simulink subsystem "HIL"  (R2024a)
settings: Solver=VariableStepAuto  StartTime=0.0  StopTime=10.0  RelTol=1e-3
values from neighbouring files (symbols this model uses):
  Hil = 100.0    [ModelDD.sldd]
  Sim : value not decoded    [ModelDD.sldd]
undefined symbols (not defined in the file or in its folder): D1, Delta, DiscIntNeverNeededParam
libraries: simulink x60, spsSeriesRLCBranchLib x18, spsControlledVoltageSourceLib x15, spsThreePhaseVIMeasurementLib x9, spsGroundLib x8, hdlsllib x6, spsMosfetLib x6, spsabctodq0Lib x5, spsDCVoltageSourceLib x3, spsPower3phInstantaneousLib x3, spsVoltageMeasurementLib x3, spspowerguiLib x3
(part 2 of 3)

== system HIL/PWM/Average ==
  DutyIn : Inport
  Iabc : Inport  Port=2
  Bias : Bias  Bias=0.5  SaturateOnIntegerOverflow=off
  Compare To Constant : simulink/Logic and Bit Operations/Compare To Constant  relop=>=  const=single(1.2)  OutDataTypeStr=boolean
  Compare To Constant1 : simulink/Logic and Bit Operations/Compare To Constant  relop=<=  const=single(0.8)  OutDataTypeStr=boolean
  Gain : Gain  Gain=-1
  Manual Switch : ManualSwitch  CurrentSetting=0
  OR : Logic  Operator=NOR  IconShape=distinctive  AllPortsSameDT=off  OutDataTypeStr=boolean
  PID Controller : slpidlib/PID Controller  Controller=PI  Form=Parallel  TimeDomain=Discrete-time  UseExternalTs=off  SampleTime=-1  IntegratorMethod=Forward Euler  FilterMethod=Forward Euler  ControllerParametersSource=internal  P=30*2/Hil.HVDC_V  I=(2*pi*4000)*30*2/Hil.HVDC_V  UseKiTs=off  D=0  UseExternalDerivativeSource=off  N=100  UseFilter=on  TunerSelectOption=Transfer Function Based (PID Tuner App)  InitialConditionSource=internal  InitialConditionForIntegrator=0  InitialConditionForFilter=0  DifferentiatorICPrevScaledInput=0  ExternalReset=none  TrackingMode=off  Kt=1  LimitOutput=on  SatLimitsSource=internal  UpperSaturationLimit=0.5  LowerSaturationLimit=-0.5  LinearizeAsGain=on  AntiWindupMode=clamping  Kb=1  LimitIntegrator=off  UpperIntegratorSaturationLimit=inf  LowerIntegratorSaturationLimit=-inf  POutMin=[]  POutMax=[]  IOutMin=[]  IOutMax=[]  DOutMin=[]  DOutMax=[]  NOutMin=[]  NOutMax=[]  SumOutMin=[]  SumOutMax=[]  SaturationOutMin=[]  SaturationOutMax=[]  PParamMin=[]  PParamMax=[]  IParamMin=[]  IParamMax=[]  DParamMin=[]  DParamMax=[]  NParamMin=[]  NParamMax=[]  KbParamMin=[]  KbParamMax=[]  KtParamMin=[]  KtParamMax=[]  KbOutMin=[]  KbOutMax=[]  KtOutMin=[]  KtOutMax=[]  IntegratorOutMin=[]  IntegratorOutMax=[]  FilterOutMin=[]  FilterOutMax=[]  SumI1OutMin=[]  SumI1OutMax=[]  SumI2OutMin=[]  SumI2OutMax=[]  SumI3OutMin=[]  SumI3OutMax=[]  SumI4OutMin=[]  SumI4OutMax=[]  SumDOutMin=[]  SumDOutMax=[]  DifferentiatorOutMin=[]  DifferentiatorOutMax=[]  FilterDiffOutCoefMin=[]  FilterDiffOutCoefMax=[]  ReciprocalOutMin=[]  ReciprocalOutMax=[]  SumDenOutMin=[]  SumDenOutMax=[]  SumNumOutMin=[]  SumNumOutMax=[]  DivideOutMin=[]  DivideOutMax=[]  UdiffTsProdOutMin=[]  UdiffTsProdOutMax=[]  NTsProdOutMin=[]  NTsProdOutMax=[]  UintegralTsProdOutMin=[]  UintegralTsProdOutMax=[]  UngainTsProdOutMin=[]  UngainTsProdOutMax=[]  ClampingZeroOutDataTypeStr=Inherit: Inherit via back propagation  ClampingZeroOutMin=[]  ClampingZeroOutMax=[]  FilterDenConstantOutDataTypeStr=Inherit: Inherit via back propagation  FilterDenConstantOutMin=[]  FilterDenConstantOutMax=[]  PCopyOutDataTypeStr=Inherit: Inherit via back propagation  PCopyOutMin=[]  PCopyOutMax=[]  NCopyOutDataTypeStr=Inherit: Inherit via back propagation  NCopyOutMin=[]  NCopyOutMax=[]  IntegratorContinuousStateAttributes=''  IntegratorStateMustResolveToSignalObject=off  IntegratorRTWStateStorageClass=Auto  FilterContinuousStateAttributes=''  FilterStateMustResolveToSignalObject=off  FilterRTWStateStorageClass=Auto  ParallelPVariant=InternalParameters  IdealPVariant=Disabled  IVariant=InternalParameters  DVariant=Disabled  IntegratorVariant=Discrete  SatVariant=Enabled  AWVariant=DiscClampingParallel  PCopyVariant=Disabled  TRVariant=Disabled  FdbkBlocksVariant=Forward  IdealPFdbkVariant=Disabled  SatFdbkVariant=Disabled  DerivativeFilterVariant=Disabled  NVariant=Disabled  NCopyVariant=Disabled_SignalSpec  FilterICVariant=Disabled  IntegratorICVariant=InternalICs  ExternalResetVariant=Disabled  TRSumVariant=Passthrough  SumFdbkVariant=Disabled  SumVariant=Sum_PI  TsampFilterVariant=InternalTs  TsampNgainVariant=Passthrough  TsampIntegralVariant=Disabled_SignalSpec  ExternalSaturationOutDataTypeStr=Inherit: Same as second input  DerivativeSourceVariant=Disabled
  Relay : Relay  OffSwitchValue=-eps  OnOutputValue=0  OffOutputValue=1
  Selector : Selector  InputPortWidth=4  IndexOptions=Index vector (dialog)  Indices=[1 2 3]  OutputSizes=1
  Selector1 : Selector  InputPortWidth=4  IndexOptions=Index vector (dialog)  Indices=[1 4]  OutputSizes=1
  Sum of Elements : Sum  Inputs=+
  Switch : Switch  Criteria=u2 > Threshold  SaturateOnIntegerOverflow=off  InputSameDT=off
  PWMSix : Outport
  wires:
  Bias/1 -> Manual Switch/2
  PID Controller/1 -> Bias/1
  Manual Switch/1 -> Switch/3
  Gain/1 -> PID Controller/1
  OR/1 -> Switch/2
  Compare To Constant1/1 -> OR/2
  Iabc/1 -> Relay/1, Gain/1
  Switch/1 -> PWMSix/1
  Selector/1 -> Switch/1
  Relay/1 -> Manual Switch/1
  DutyIn/1 -> Selector1/1, Selector/1  "HIL_PWM"
  Selector1/1 -> Sum of Elements/1
  Sum of Elements/1 -> Compare To Constant/1, Compare To Constant1/1
  Compare To Constant/1 -> OR/1

== system HIL/PWM/PWM ==
  DutyIn : Inport
  Compare To Constant : simulink/Logic and Bit Operations/Compare To Constant  relop=<=  const=0.5  OutDataTypeStr=boolean
  Constant : Constant  Value=round(1/(Hil.PWM_Freq*Sim.ContSampleTime))
  Constant1 : Constant  OutDataTypeStr=boolean
  Constant2 : Constant  Value=round(Hil.PWM_Deadtime/Sim.ContSampleTime)  OutDataTypeStr=uint32
  Gain2 : Gain  Gain=0.5  OutDataTypeStr=uint32
  NOT : Logic  Operator=NOT  IconShape=distinctive  AllPortsSameDT=off  OutDataTypeStr=boolean
  PWM Generator : Subsystem
  Product : Product
  Product1 : Product
  Selector2 : Selector  InputPortWidth=4  IndexOptions=Index vector (dialog)  Indices=[1 2 3]  OutputSizes=1
  Selector3 : Selector  InputPortWidth=4  IndexOptions=Index vector (dialog)  Indices=[1 4]  OutputSizes=1
  Sum of Elements : Sum  Inputs=+
  Unit Delay1 : UnitDelay  SampleTime=-1  HasFrameUpgradeWarning=on
  PWMSix : Outport
  Trig : Outport  Port=2
  wires:
  DutyIn/1 -> Selector2/1, Selector3/1  "DutyIn"
  Sum of Elements/1 -> Compare To Constant/1
  Selector3/1 -> Sum of Elements/1  "DutyIn"
  Selector2/1 -> Product/1  "DutyIn"
  Compare To Constant/1 -> Unit Delay1/1
  PWM Generator/1(S) -> Product1/2
  Gain2/1 -> PWM Generator/2(Period), Product/2
  Constant1/1 -> PWM Generator/3(Enable)
  Constant2/1 -> PWM Generator/4(DeadBand)
  Constant/1 -> Gain2/1
  Product/1 -> PWM Generator/1(DutyCnt)  "DutyCnt"
  PWM Generator/2(Trig) -> Trig/1
  Unit Delay1/1 -> NOT/1
  Product1/1 -> PWMSix/1
  NOT/1 -> Product1/1

== system HIL/Sensors/Delta ==
  Vabc_g : Inport
  Iabc : Inport  Port=2
  Vdc : Inport  Port=3
  Bias : Bias  Bias=Hil.ADC_CH0_PHY_OFFSET  SaturateOnIntegerOverflow=off
  Bias1 : Bias  Bias=Hil.ADC_CH1_PHY_OFFSET  SaturateOnIntegerOverflow=off
  Bias2 : Bias  Bias=Hil.ADC_CH2_PHY_OFFSET  SaturateOnIntegerOverflow=off
  Bias3 : Bias  Bias=Hil.ADC_CH3_PHY_OFFSET  SaturateOnIntegerOverflow=off
  Bias4 : Bias  Bias=Hil.ADC_CH4_PHY_OFFSET  SaturateOnIntegerOverflow=off
  Bias5 : Bias  Bias=Hil.ADC_CH5_PHY_OFFSET  SaturateOnIntegerOverflow=off
  Demux2 : Demux  Outputs=3
  Demux3 : Demux  Outputs=3
  Gain : Gain  Gain=1/Hil.ADC_CH0_PHY_Gain
  Gain1 : Gain  Gain=1/Hil.ADC_CH4_PHY_Gain
  Gain2 : Gain  Gain=1/Hil.ADC_CH1_PHY_Gain
  Gain3 : Gain  Gain=1/Hil.ADC_CH3_PHY_Gain
  Gain5 : Gain  Gain=1/Hil.ADC_CH2_PHY_Gain
  Gain6 : Gain  Gain=1/Hil.ADC_CH5_PHY_Gain
  Terminator : Terminator
  ADC1 : Outport
  ADC2 : Outport  Port=2
  ADC3 : Outport  Port=3
  ADC4 : Outport  Port=4
  ADC5 : Outport  Port=5
  ADC6 : Outport  Port=6
  wires:
  Gain1/1 -> Bias4/1
  Gain5/1 -> Bias2/1
  Demux2/2 -> Gain2/1
  Demux2/1 -> Gain/1
  Gain6/1 -> Bias5/1
  Gain/1 -> Bias/1
  Demux3/1 -> Gain5/1
  Demux3/3 -> Gain1/1
  Gain3/1 -> Bias3/1
  Bias5/1 -> ADC6/1  "V_hvdc_5v"
  Bias1/1 -> ADC2/1  "V_Grid_b_5v"
  Demux3/2 -> Gain3/1
  Gain2/1 -> Bias1/1
  Iabc/1 -> Demux3/1
  Vabc_g/1 -> Demux2/1
  Bias/1 -> ADC1/1  "V_Grid_a_5v"
  Bias4/1 -> ADC5/1  "I_inv_b_5v"
  Bias2/1 -> ADC3/1  "V_Grid_c_5v"
  Vdc/1 -> Gain6/1
  Bias3/1 -> ADC4/1  "I_inv_a_5v"
  Demux2/3 -> Terminator/1

== system HIL/Sensors/Star ==
  Vabc_g : Inport
  Iabc : Inport  Port=2
  Vdc : Inport  Port=3
  Bias : Bias  Bias=Hil.ADC_CH0_PHY_OFFSET  SaturateOnIntegerOverflow=off
  Bias1 : Bias  Bias=Hil.ADC_CH1_PHY_OFFSET  SaturateOnIntegerOverflow=off
  Bias2 : Bias  Bias=Hil.ADC_CH2_PHY_OFFSET  SaturateOnIntegerOverflow=off
  Bias3 : Bias  Bias=Hil.ADC_CH3_PHY_OFFSET  SaturateOnIntegerOverflow=off
  Bias4 : Bias  Bias=Hil.ADC_CH4_PHY_OFFSET  SaturateOnIntegerOverflow=off
  Bias5 : Bias  Bias=Hil.ADC_CH5_PHY_OFFSET  SaturateOnIntegerOverflow=off
  Demux2 : Demux  Outputs=3
  Demux3 : Demux  Outputs=3
  Gain : Gain  Gain=1/Hil.ADC_CH0_PHY_Gain
  Gain1 : Gain  Gain=1/Hil.ADC_CH4_PHY_Gain
  Gain2 : Gain  Gain=1/Hil.ADC_CH1_PHY_Gain
  Gain3 : Gain  Gain=1/Hil.ADC_CH3_PHY_Gain
  Gain5 : Gain  Gain=1/Hil.ADC_CH2_PHY_Gain
  Gain6 : Gain  Gain=1/Hil.ADC_CH5_PHY_Gain
  Terminator1 : Terminator
  ADC1 : Outport
  ADC2 : Outport  Port=2
  ADC3 : Outport  Port=3
  ADC4 : Outport  Port=4
  ADC5 : Outport  Port=5
  ADC6 : Outport  Port=6
  wires:
  Bias3/1 -> ADC4/1  "I_inv_a_5v"
  Vdc/1 -> Gain6/1
  Bias2/1 -> ADC3/1  "V_Grid_c_5v"
  Bias4/1 -> ADC5/1  "I_inv_b_5v"
  Bias/1 -> ADC1/1  "V_Grid_a_5v"
  Vabc_g/1 -> Demux2/1
  Iabc/1 -> Demux3/1
  Gain2/1 -> Bias1/1
  Demux3/3 -> Terminator1/1
  Demux3/1 -> Gain3/1
  Bias1/1 -> ADC2/1  "V_Grid_b_5v"
  Bias5/1 -> ADC6/1  "V_hvdc_5v"
  Gain3/1 -> Bias3/1
  Demux3/2 -> Gain1/1
  Demux2/3 -> Gain5/1
  Gain/1 -> Bias/1
  Gain6/1 -> Bias5/1
  Demux2/1 -> Gain/1
  Demux2/2 -> Gain2/1
  Gain5/1 -> Bias2/1
  Gain1/1 -> Bias4/1

== system HIL/EquivelentSimscape/Continous/Harmonics ==
  wt_abc : Inport
  Enable : EnablePort
  Cos1 : Trigonometry  Operator=cos
  Gain5 : Gain  Gain=Hil.Harm_Freq'  Multiplication=Matrix(K*u)
  Gain8 : Gain  Gain=(eye(3,3).*(Hil.Harm_Amp))  Multiplication=Matrix(K*u)
  Reshape : Reshape
  Reshape1 : Reshape  OutputDimensionality=Row vector (2-D)
  Sum of Elements : Sum  Inputs=+  CollapseMode=Specified dimension
  Harm : Outport
  wires:
  Reshape/1 -> Harm/1
  Gain8/1 -> Sum of Elements/1
  Cos1/1 -> Gain8/1
  Gain5/1 -> Cos1/1
  Reshape1/1 -> Gain5/1
  wt_abc/1 -> Reshape1/1
  Sum of Elements/1 -> Reshape/1

== system HIL/EquivelentSimscape/Continous/Phase2Line ==
  In1 : Inport
  Demux : Demux  Outputs=3
  Mux1 : Mux  Inputs=3
  Sum{,1..3} (4 alike) : Sum  Inputs=|+-
  Sum4 : Sum  Inputs=-+|
  Sum5 : Sum  Inputs=-+|
  Out1 : Outport
  wires:
  Sum2/1 -> Sum5/2, Sum3/2  "CA"
  Sum1/1 -> Sum4/2, Sum5/1  "BC"
  Sum4/1 -> Mux1/2  "BC-AB"
  Sum5/1 -> Mux1/3  "CA-BC"
  Mux1/1 -> Out1/1
  Sum3/1 -> Mux1/1  "AB-CA"
  Sum/1 -> Sum3/1, Sum4/1  "AB"
  Demux/1 -> Sum/1, Sum2/2  "A"
  Demux/2 -> Sum1/1, Sum/2  "B"
  In1/1 -> Demux/1
  Demux/3 -> Sum2/1, Sum1/2  "C"

== system HIL/EquivelentSimscape/Continous/Phase2Line1 ==
  In1 : Inport
  Demux : Demux  Outputs=3
  Mux1 : Mux  Inputs=3
  Sum{,1..3} (4 alike) : Sum  Inputs=|+-
  Sum4 : Sum  Inputs=-+|
  Sum5 : Sum  Inputs=-+|
  Out1 : Outport
  wires:
  Demux/3 -> Sum1/2, Sum2/1  "C"
  In1/1 -> Demux/1
  Demux/2 -> Sum/2, Sum1/1  "B"
  Demux/1 -> Sum2/2, Sum/1  "A"
  Sum/1 -> Sum4/1, Sum3/1  "AB"
  Sum3/1 -> Mux1/1  "AB-CA"
  Mux1/1 -> Out1/1
  Sum5/1 -> Mux1/3  "CA-BC"
  Sum4/1 -> Mux1/2  "BC-AB"
  Sum1/1 -> Sum5/1, Sum4/2  "BC"
  Sum2/1 -> Sum3/2, Sum5/2  "CA"

== system HIL/EquivelentSimscape/Continous/Rectifier1 ==
  Io : Inport
  Abs : Abs  SaturateOnIntegerOverflow=off
  Constant : Constant  Value=Hil.Grid_Frq
  Cos : Trigonometry  Operator=cos
  Discrete-Time Integrator : DiscreteIntegrator  gainval=single(1)  InitialCondition=single(311)  SampleTime=-1  ICPrevOutput=DiscIntNeverNeededParam  ICPrevScaledInput=DiscIntNeverNeededParam
  Gain : Gain  Gain=1/Hil.HVDC_C
  Gain1 : Gain  Gain=1/0.2
  Gain2 : Gain  Gain=2*pi
  Gain3 : Gain  Gain=Hil.Grid_VphRms*sqrt(2)
  Gain4 : Gain  Gain=Hil.HVDC_Cesr
  Gain5 : Gain  Gain=1/500
  Gain6 : Gain  Gain=Hil.HVDC_AutoTrnsN
  Saturation : Saturate  UpperLimit=inf  LowerLimit=0
  Sum : Sum  Inputs=|++
  Sum1 : Sum  Inputs=-+-
  Sum2 : Sum  Inputs=|+-
  Unit Delay1 : UnitDelay  InitialCondition=single(311)  SampleTime=-1  HasFrameUpgradeWarning=on
  Unit Delay2 : UnitDelay  SampleTime=-1  HasFrameUpgradeWarning=on
  WrappedIntegrator : Subsystem
  Vo : Outport
  wires:
  Gain6/1 -> Abs/1  "Vrec"
  Gain5/1 -> Sum1/3
  Gain4/1 -> Sum/2
  Discrete-Time Integrator/1 -> Sum/1
  Abs/1 -> Sum2/1  "Vrec"
  Sum/1 -> Vo/1, Unit Delay1/1  "Vdc"
  Sum1/1 -> Gain/1, Gain4/1  "Ic"
  Gain/1 -> Discrete-Time Integrator/1
  Unit Delay1/1 -> Sum2/2, Gain5/1
  Saturation/1 -> Sum1/2
  Unit Delay2/1 -> Sum1/1
  Io/1 -> Unit Delay2/1
  Sum2/1 -> Gain1/1
  Gain3/1 -> Gain6/1  "Vrec"
  Gain1/1 -> Saturation/1  "ir"
  WrappedIntegrator/1(wt) -> Cos/1  "wt"
  Gain2/1 -> WrappedIntegrator/1(w)  "w"
  Cos/1 -> Gain3/1
  Constant/1 -> Gain2/1  "f"

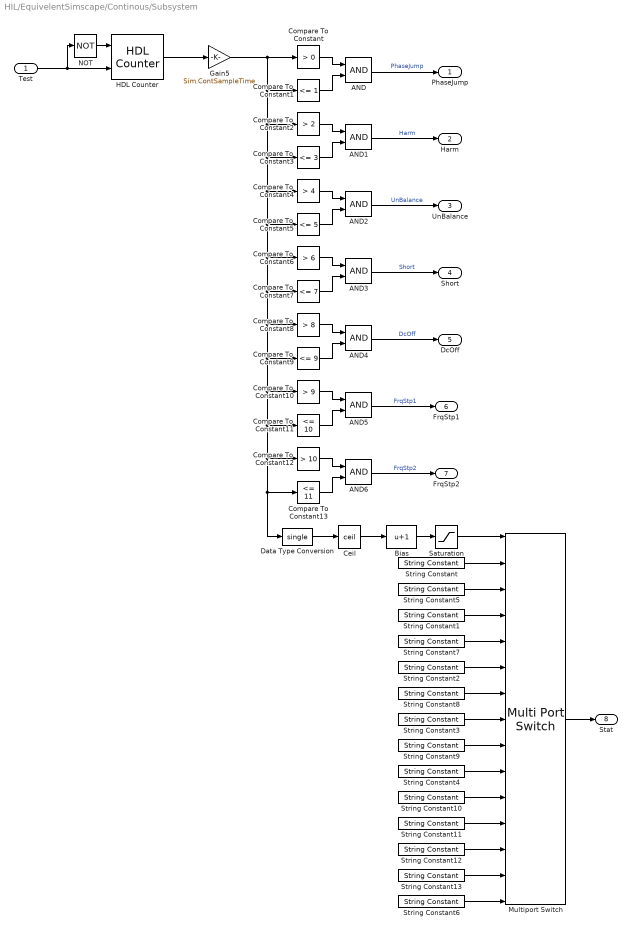
== system HIL/EquivelentSimscape/Continous/Subsystem ==
  Test : Inport
  AND{,1..6} (7 alike) : Logic  AllPortsSameDT=off  OutDataTypeStr=boolean
  Bias : Bias  Bias=1  SaturateOnIntegerOverflow=off
  Ceil : Rounding  Operator=ceil
  Compare To Constant : simulink/Logic and Bit Operations/Compare To Constant  relop=>  const=0  OutDataTypeStr=boolean
  Compare To Constant1 : simulink/Logic and Bit Operations/Compare To Constant  relop=<=  const=1  OutDataTypeStr=boolean
  Compare To Constant10 : simulink/Logic and Bit Operations/Compare To Constant  relop=>  const=9  OutDataTypeStr=boolean
  Compare To Constant11 : simulink/Logic and Bit Operations/Compare To Constant  relop=<=  const=10  OutDataTypeStr=boolean
  Compare To Constant12 : simulink/Logic and Bit Operations/Compare To Constant  relop=>  const=10  OutDataTypeStr=boolean
  Compare To Constant13 : simulink/Logic and Bit Operations/Compare To Constant  relop=<=  const=11  OutDataTypeStr=boolean
  Compare To Constant2 : simulink/Logic and Bit Operations/Compare To Constant  relop=>  const=2  OutDataTypeStr=boolean
  Compare To Constant3 : simulink/Logic and Bit Operations/Compare To Constant  relop=<=  const=3  OutDataTypeStr=boolean
  Compare To Constant4 : simulink/Logic and Bit Operations/Compare To Constant  relop=>  const=4  OutDataTypeStr=boolean
  Compare To Constant5 : simulink/Logic and Bit Operations/Compare To Constant  relop=<=  const=5  OutDataTypeStr=boolean
  Compare To Constant6 : simulink/Logic and Bit Operations/Compare To Constant  relop=>  const=6  OutDataTypeStr=boolean
  Compare To Constant7 : simulink/Logic and Bit Operations/Compare To Constant  relop=<=  const=7  OutDataTypeStr=boolean
  Compare To Constant8 : simulink/Logic and Bit Operations/Compare To Constant  relop=>  const=8  OutDataTypeStr=boolean
  Compare To Constant9 : simulink/Logic and Bit Operations/Compare To Constant  relop=<=  const=9  OutDataTypeStr=boolean
  Data Type Conversion : DataTypeConversion  OutDataTypeStr=single  SaturateOnIntegerOverflow=off  RndMeth=Floor
  Gain5 : Gain  Gain=Sim.ContSampleTime  ParamDataTypeStr=double  OutDataTypeStr=double
  HDL Counter : hdlsllib/Sources/HDL Counter  CountType=Free running  CountInit=0  CountStep=1  CountMax=25  CountFromType=Initial value  CountFrom=0  CountResetPort=on  CountLoadPort=off  CountEnbPort=on  CountDirPort=off  CountHitOutputPort=off  CountDataType=Unsigned  CountWordLen=32  CountFracLen=0  CountSampTime=1
  Multiport Switch : MultiPortSwitch  Inputs=14  SaturateOnIntegerOverflow=off  InputSameDT=off
  NOT : Logic  Operator=NOT  AllPortsSameDT=off  OutDataTypeStr=boolean
  Saturation : Saturate  UpperLimit=14  LowerLimit=0
  String Constant{,1..4,6,11} (7 alike) : StringConstant  String="\"Normal\""
  String Constant10 : StringConstant  String="\"DC Offset\""
  String Constant12 : StringConstant  String="\"Freq Stp 1\""
  String Constant13 : StringConstant  String="\"Freq Stp 2\""
  String Constant5 : StringConstant  String="\"Phase Jump\""
  String Constant7 : StringConstant  String="\"Harm\""
  String Constant8 : StringConstant  String="\"Unbalance\""
  String Constant9 : StringConstant  String="\"Short\""
  PhaseJump : Outport
  Harm : Outport  Port=2
  UnBalance : Outport  Port=3
  Short : Outport  Port=4
  DcOff : Outport  Port=5
  FrqStp1 : Outport  Port=6
  FrqStp2 : Outport  Port=7
  Stat : Outport  Port=8
  wires:
  Bias/1 -> Saturation/1
  Data Type Conversion/1 -> Ceil/1
  Multiport Switch/1 -> Stat/1
  Saturation/1 -> Multiport Switch/1
  Ceil/1 -> Bias/1
  String Constant13/1 -> Multiport Switch/14
  String Constant12/1 -> Multiport Switch/13
  String Constant11/1 -> Multiport Switch/12
  String Constant10/1 -> Multiport Switch/11
  String Constant9/1 -> Multiport Switch/9
  String Constant8/1 -> Multiport Switch/7
  String Constant7/1 -> Multiport Switch/5
  String Constant5/1 -> Multiport Switch/3
  String Constant6/1 -> Multiport Switch/15
  String Constant4/1 -> Multiport Switch/10
  String Constant3/1 -> Multiport Switch/8
  String Constant2/1 -> Multiport Switch/6
  String Constant1/1 -> Multiport Switch/4
  String Constant/1 -> Multiport Switch/2
  NOT/1 -> HDL Counter/1
  Compare To Constant13/1 -> AND6/2
  Compare To Constant12/1 -> AND6/1
  AND6/1 -> FrqStp2/1  "FrqStp2"
  AND5/1 -> FrqStp1/1  "FrqStp1"
  Compare To Constant10/1 -> AND5/1
  Compare To Constant11/1 -> AND5/2
  AND/1 -> PhaseJump/1  "PhaseJump"
  Test/1 -> HDL Counter/2, NOT/1
  AND2/1 -> UnBalance/1  "UnBalance"
  AND3/1 -> Short/1  "Short"
  HDL Counter/1 -> Gain5/1
  Compare To Constant5/1 -> AND2/2
  Compare To Constant/1 -> AND/1
  Compare To Constant9/1 -> AND4/2
  Compare To Constant2/1 -> AND1/1
  Compare To Constant8/1 -> AND4/1
  Compare To Constant3/1 -> AND1/2
  AND4/1 -> DcOff/1  "DcOff"
  Compare To Constant1/1 -> AND/2
  Compare To Constant7/1 -> AND3/2
  Compare To Constant6/1 -> AND3/1
  Gain5/1 -> Compare To Constant/1, Compare To Constant1/1, Compare To Constant3/1, Compare To Constant5/1, Compare To Constant7/1, Compare To Constant8/1, Compare To Constant9/1, Compare To Constant13/1, Data Type Conversion/1, Compare To Constant12/1, Compare To Constant11/1, Compare To Constant10/1, Compare To Constant6/1, Compare To Constant4/1, Compare To Constant2/1
  AND1/1 -> Harm/1  "Harm"
  Compare To Constant4/1 -> AND2/1

== system HIL/EquivelentSimscape/Continous/WrappedIntegrator ==
  w : Inport
  Constant1 : Constant  Value=2*pi
  Discrete-Time Integrator1 : DiscreteIntegrator  gainval=single(1)  ExternalReset=rising  InitialConditionSource=external  SampleTime=-1  ShowStatePort=on  ICPrevOutput=DiscIntNeverNeededParam  ICPrevScaledInput=DiscIntNeverNeededParam
  GreaterThan : RelationalOperator  Operator=~=  OutDataTypeStr=boolean  RndMeth=Simplest  InputSameDT=off
  Mod : Math  Operator=mod
  wt : Outport
  wires:
  GreaterThan/1 -> Discrete-Time Integrator1/2
  Discrete-Time Integrator1/1 -> wt/1  "wt"
  w/1 -> Discrete-Time Integrator1/1
  Discrete-Time Integrator1/State -> Mod/1, GreaterThan/1
  Mod/1 -> GreaterThan/2, Discrete-Time Integrator1/3
  Constant1/1 -> Mod/2

== system HIL/EquivelentSimscape/Continous/abc_dqz ==
  abc : Inport
  Ang : Inport  Port=2
  Subsystem : Subsystem
  Subsystem2 : Subsystem
  dqz : Outport  VectorParamsAs1DForOutWhenUnconnected=off
  wires:
  Subsystem2/1(dq) -> dqz/1
  Ang/1 -> Subsystem2/2(wtNow)
  Subsystem/1(al_be_0) -> Subsystem2/1(alpha_beta)
  abc/1 -> Subsystem/1(abc)

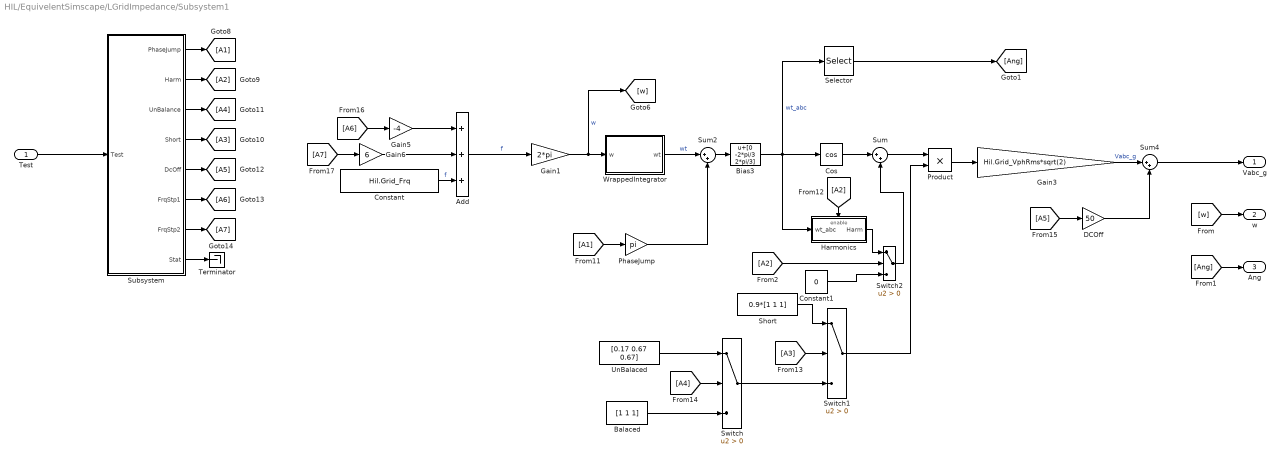
== system HIL/EquivelentSimscape/LGridImpedance/Subsystem1 ==
  Test : Inport
  Add : Sum  Inputs=+++
  Balaced : Constant  Value=[1 1 1]
  Bias3 : Bias  Bias=[0 -2*pi/3 2*pi/3]  SaturateOnIntegerOverflow=off
  Constant : Constant  Value=Hil.Grid_Frq
  Constant1 : Constant  Value=0
  Cos : Trigonometry  Operator=cos
  DCOff : Gain  Gain=50
  Gain1 : Gain  Gain=2*pi
  Gain3 : Gain  Gain=Hil.Grid_VphRms*sqrt(2)
  Gain5 : Gain  Gain=-4
  Gain6 : Gain  Gain=6
  Harmonics : Subsystem
  PhaseJump : Gain  Gain=pi
  Product : Product
  Selector : Selector  InputPortWidth=3  IndexOptions=Index vector (dialog)  Indices=[1]  OutputSizes=1
  Short : Constant  Value=0.9*[1 1 1]
  Subsystem : Subsystem
  Sum : Sum  Inputs=|++
  Sum2 : Sum  Inputs=|++
  Sum4 : Sum  Inputs=|++
  Switch : Switch  Criteria=u2 > Threshold  SaturateOnIntegerOverflow=off  InputSameDT=off
  Switch1 : Switch  Criteria=u2 > Threshold  SaturateOnIntegerOverflow=off  InputSameDT=off
  Switch2 : Switch  Criteria=u2 > Threshold  SaturateOnIntegerOverflow=off  InputSameDT=off
  Terminator : Terminator
  UnBalaced : Constant  Value=[0.17 0.67 0.67]
  WrappedIntegrator : Subsystem
  Vabc_g : Outport
  w : Outport  Port=2
  Ang : Outport  Port=3
  wires:
  [A2] -> Switch2/2
  Constant1/1 -> Switch2/3
  Harmonics/1(Harm) -> Switch2/1
  Subsystem/1(PhaseJump) -> [A1]
  [w] -> w/1
  [Ang] -> Ang/1
  Balaced/1 -> Switch/3
  Sum4/1 -> Vabc_g/1
  Test/1 -> Subsystem/1(Test)
  Cos/1 -> Sum/1
  Gain1/1 -> WrappedIntegrator/1(w), [w]  "w"
  Add/1 -> Gain1/1  "f"
  Selector/1 -> [Ang]
  PhaseJump/1 -> Sum2/2
  Gain3/1 -> Sum4/1  "Vabc_g"
  [A3] -> Switch1/2
  Subsystem/5(DcOff) -> [A5]
  Product/1 -> Gain3/1
  [A2] -> Harmonics/Enable
  Switch/1 -> Switch1/3
  Short/1 -> Switch1/1
  [A4] -> Switch/2
  Sum/1 -> Product/1
  Constant/1 -> Add/3  "f"
  Gain6/1 -> Add/2
  Subsystem/2(Harm) -> [A2]
  DCOff/1 -> Sum4/2
  Switch1/1 -> Product/2
  [A7] -> Gain6/1
  Subsystem/6(FrqStp1) -> [A6]
  WrappedIntegrator/1(wt) -> Sum2/1  "wt"
  Subsystem/8(Stat) -> Terminator/1
  [A6] -> Gain5/1
  UnBalaced/1 -> Switch/1
  Sum2/1 -> Bias3/1
  Gain5/1 -> Add/1
  [A5] -> DCOff/1
  Subsystem/7(FrqStp2) -> [A7]
  [A1] -> PhaseJump/1
  Bias3/1 -> Harmonics/1(wt_abc), Selector/1, Cos/1  "wt_abc"
  Switch2/1 -> Sum/2
  Subsystem/4(Short) -> [A3]
  Subsystem/3(UnBalance) -> [A4]

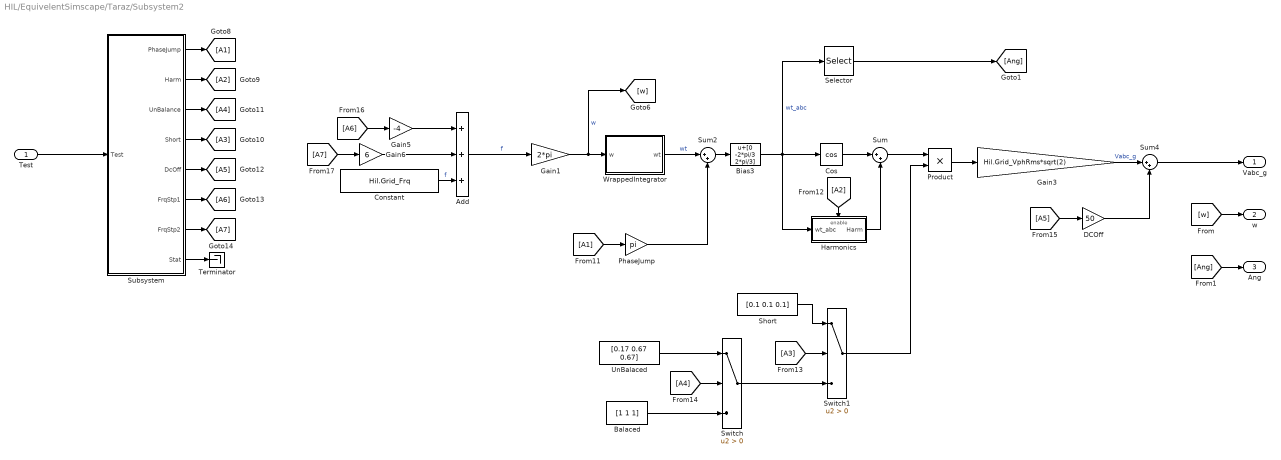
== system HIL/EquivelentSimscape/Taraz/Subsystem2 ==
  Test : Inport
  Add : Sum  Inputs=+++
  Balaced : Constant  Value=[1 1 1]
  Bias3 : Bias  Bias=[0 -2*pi/3 2*pi/3]  SaturateOnIntegerOverflow=off
  Constant : Constant  Value=Hil.Grid_Frq
  Cos : Trigonometry  Operator=cos
  DCOff : Gain  Gain=50
  Gain1 : Gain  Gain=2*pi
  Gain3 : Gain  Gain=Hil.Grid_VphRms*sqrt(2)
  Gain5 : Gain  Gain=-4
  Gain6 : Gain  Gain=6
  Harmonics : Subsystem
  PhaseJump : Gain  Gain=pi
  Product : Product
  Selector : Selector  InputPortWidth=3  IndexOptions=Index vector (dialog)  Indices=[1]  OutputSizes=1
  Short : Constant  Value=[0.1 0.1 0.1]
  Subsystem : Subsystem
  Sum : Sum  Inputs=|++
  Sum2 : Sum  Inputs=|++
  Sum4 : Sum  Inputs=|++
  Switch : Switch  Criteria=u2 > Threshold  SaturateOnIntegerOverflow=off  InputSameDT=off
  Switch1 : Switch  Criteria=u2 > Threshold  SaturateOnIntegerOverflow=off  InputSameDT=off
  Terminator : Terminator
  UnBalaced : Constant  Value=[0.17 0.67 0.67]
  WrappedIntegrator : Subsystem
  Vabc_g : Outport
  w : Outport  Port=2
  Ang : Outport  Port=3
  wires:
  Subsystem/1(PhaseJump) -> [A1]
  [w] -> w/1
  [Ang] -> Ang/1
  Balaced/1 -> Switch/3
  Sum4/1 -> Vabc_g/1
  Test/1 -> Subsystem/1(Test)
  Cos/1 -> Sum/1
  Gain1/1 -> WrappedIntegrator/1(w), [w]  "w"
  Add/1 -> Gain1/1  "f"
  Selector/1 -> [Ang]
  PhaseJump/1 -> Sum2/2
  Gain3/1 -> Sum4/1  "Vabc_g"
  [A3] -> Switch1/2
  Subsystem/5(DcOff) -> [A5]
  Product/1 -> Gain3/1
  [A2] -> Harmonics/Enable
  Switch/1 -> Switch1/3
  Short/1 -> Switch1/1
  [A4] -> Switch/2
  Sum/1 -> Product/1
  Constant/1 -> Add/3  "f"
  Gain6/1 -> Add/2
  Subsystem/2(Harm) -> [A2]
  DCOff/1 -> Sum4/2
  Switch1/1 -> Product/2
  [A7] -> Gain6/1
  Subsystem/6(FrqStp1) -> [A6]
  WrappedIntegrator/1(wt) -> Sum2/1  "wt"
  Subsystem/8(Stat) -> Terminator/1
  [A6] -> Gain5/1
  UnBalaced/1 -> Switch/1
  Sum2/1 -> Bias3/1
  Gain5/1 -> Add/1
  [A5] -> DCOff/1
  Subsystem/7(FrqStp2) -> [A7]
  [A1] -> PhaseJump/1
  Bias3/1 -> Harmonics/1(wt_abc), Selector/1, Cos/1  "wt_abc"
  Harmonics/1(Harm) -> Sum/2
  Subsystem/4(Short) -> [A3]
  Subsystem/3(UnBalance) -> [A4]

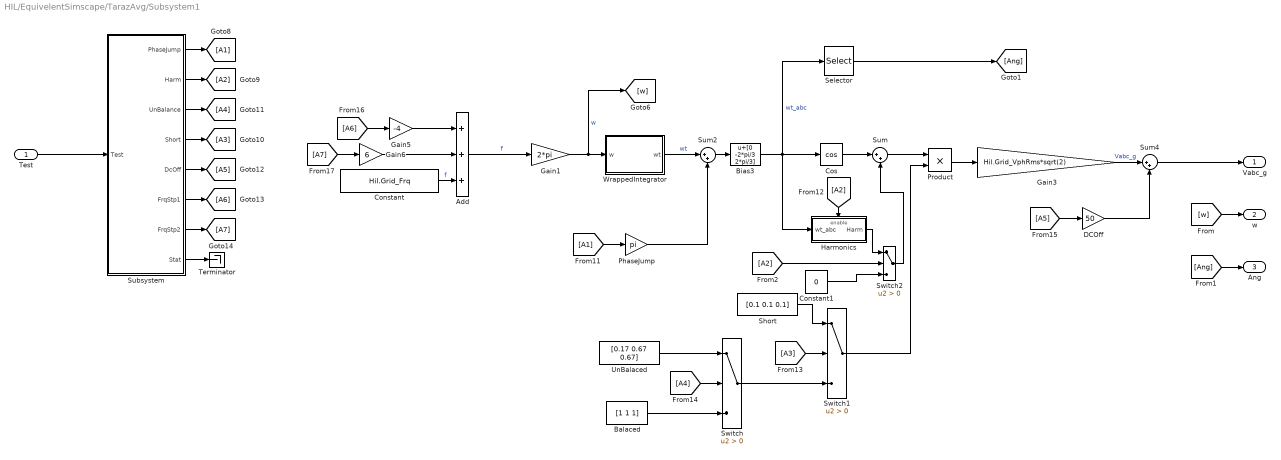
== system HIL/EquivelentSimscape/TarazAvg/Subsystem1 ==
  Test : Inport
  Add : Sum  Inputs=+++
  Balaced : Constant  Value=[1 1 1]
  Bias3 : Bias  Bias=[0 -2*pi/3 2*pi/3]  SaturateOnIntegerOverflow=off
  Constant : Constant  Value=Hil.Grid_Frq
  Constant1 : Constant  Value=0
  Cos : Trigonometry  Operator=cos
  DCOff : Gain  Gain=50
  Gain1 : Gain  Gain=2*pi
  Gain3 : Gain  Gain=Hil.Grid_VphRms*sqrt(2)
  Gain5 : Gain  Gain=-4
  Gain6 : Gain  Gain=6
  Harmonics : Subsystem
  PhaseJump : Gain  Gain=pi
  Product : Product
  Selector : Selector  InputPortWidth=3  IndexOptions=Index vector (dialog)  Indices=[1]  OutputSizes=1
  Short : Constant  Value=[0.1 0.1 0.1]
  Subsystem : Subsystem
  Sum : Sum  Inputs=|++
  Sum2 : Sum  Inputs=|++
  Sum4 : Sum  Inputs=|++
  Switch : Switch  Criteria=u2 > Threshold  SaturateOnIntegerOverflow=off  InputSameDT=off
  Switch1 : Switch  Criteria=u2 > Threshold  SaturateOnIntegerOverflow=off  InputSameDT=off
  Switch2 : Switch  Criteria=u2 > Threshold  SaturateOnIntegerOverflow=off  InputSameDT=off
  Terminator : Terminator
  UnBalaced : Constant  Value=[0.17 0.67 0.67]
  WrappedIntegrator : Subsystem
  Vabc_g : Outport
  w : Outport  Port=2
  Ang : Outport  Port=3
  wires:
  [A2] -> Switch2/2
  Constant1/1 -> Switch2/3
  Harmonics/1(Harm) -> Switch2/1
  Subsystem/1(PhaseJump) -> [A1]
  [w] -> w/1
  [Ang] -> Ang/1
  Balaced/1 -> Switch/3
  Sum4/1 -> Vabc_g/1
  Test/1 -> Subsystem/1(Test)
  Cos/1 -> Sum/1
  Gain1/1 -> WrappedIntegrator/1(w), [w]  "w"
  Add/1 -> Gain1/1  "f"
  Selector/1 -> [Ang]
  PhaseJump/1 -> Sum2/2
  Gain3/1 -> Sum4/1  "Vabc_g"
  [A3] -> Switch1/2
  Subsystem/5(DcOff) -> [A5]
  Product/1 -> Gain3/1
  [A2] -> Harmonics/Enable
  Switch/1 -> Switch1/3
  Short/1 -> Switch1/1
  [A4] -> Switch/2
  Sum/1 -> Product/1
  Constant/1 -> Add/3  "f"
  Gain6/1 -> Add/2
  Subsystem/2(Harm) -> [A2]
  DCOff/1 -> Sum4/2
  Switch1/1 -> Product/2
  [A7] -> Gain6/1
  Subsystem/6(FrqStp1) -> [A6]
  WrappedIntegrator/1(wt) -> Sum2/1  "wt"
  Subsystem/8(Stat) -> Terminator/1
  [A6] -> Gain5/1
  UnBalaced/1 -> Switch/1
  Sum2/1 -> Bias3/1
  Gain5/1 -> Add/1
  [A5] -> DCOff/1
  Subsystem/7(FrqStp2) -> [A7]
  [A1] -> PhaseJump/1
  Bias3/1 -> Harmonics/1(wt_abc), Selector/1, Cos/1  "wt_abc"
  Switch2/1 -> Sum/2
  Subsystem/4(Short) -> [A3]
  Subsystem/3(UnBalance) -> [A4]

== system HIL/PWM/PWM/PWM Generator ==
  DutyCnt : Inport
  Period : Inport  Port=2
  Enable : Inport  Port=3
  DeadBand : Inport  Port=4
  AND : Logic  AllPortsSameDT=off  OutDataTypeStr=boolean
  Add : Sum
  Carrier : Subsystem
  Demux : Demux  Outputs=3
  Mux : Mux  Inputs=6
  Relational Operator : RelationalOperator  Operator=<=  OutDataTypeStr=boolean  InputSameDT=off
  Relational Operator1 : RelationalOperator  Operator=<=  OutDataTypeStr=boolean  InputSameDT=off
  Relational Operator2 : RelationalOperator  Operator=<=  OutDataTypeStr=boolean  InputSameDT=off
  Relational Operator3 : RelationalOperator  Operator=>  OutDataTypeStr=boolean  InputSameDT=off
  Relational Operator4 : RelationalOperator  Operator=>  OutDataTypeStr=boolean  InputSameDT=off
  Relational Operator5 : RelationalOperator  Operator=>  OutDataTypeStr=boolean  InputSameDT=off
  Unit Delay{,1..4} (5 alike) : UnitDelay  SampleTime=-1  HasFrameUpgradeWarning=on
  S : Outport  VectorParamsAs1DForOutWhenUnconnected=off
  Trig : Outport  Port=2  VectorParamsAs1DForOutWhenUnconnected=off
  wires:
  Period/1 -> Unit Delay1/1
  Mux/1 -> AND/1  "G"
  Enable/1 -> Unit Delay2/1
  Relational Operator5/1 -> Mux/6  "C_"
  Relational Operator2/1 -> Mux/5  "C"
  Relational Operator3/1 -> Mux/2  "A_"
  DutyCnt/1 -> Unit Delay/1
  Relational Operator4/1 -> Mux/4  "B_"
  Relational Operator/1 -> Mux/1  "A"
  Relational Operator1/1 -> Mux/3  "B"
  Demux/1 -> Relational Operator3/2, Relational Operator/2  "A_comp"
  Demux/2 -> Relational Operator4/2, Relational Operator1/2  "B_comp"
  Demux/3 -> Relational Operator5/2, Relational Operator2/2  "C_comp"
  DeadBand/1 -> Unit Delay3/1
  Add/1 -> Relational Operator2/1, Relational Operator1/1, Relational Operator/1
  Unit Delay/1 -> Demux/1
  Unit Delay1/1 -> Carrier/2(PWM Period)
  Unit Delay2/1 -> AND/2, Carrier/1(Enable)
  Unit Delay3/1 -> Add/1  "Deadtime_Cnt"
  Unit Delay4/1 -> S/1  "PWM_T_abc"
  AND/1 -> Unit Delay4/1
  Carrier/1(Counter) -> Add/2, Relational Operator3/1, Relational Operator4/1, Relational Operator5/1
  Carrier/2(Trig) -> Trig/1

== system HIL/EquivelentSimscape/Continous/Rectifier1/WrappedIntegrator ==
  w : Inport
  Constant1 : Constant  Value=2*pi
  Discrete-Time Integrator1 : DiscreteIntegrator  gainval=single(1)  ExternalReset=rising  InitialConditionSource=external  SampleTime=-1  ShowStatePort=on  ICPrevOutput=DiscIntNeverNeededParam  ICPrevScaledInput=DiscIntNeverNeededParam
  GreaterThan : RelationalOperator  Operator=~=  OutDataTypeStr=boolean  RndMeth=Simplest  InputSameDT=off
  Mod : Math  Operator=mod
  wt : Outport
  wires:
  Constant1/1 -> Mod/2
  Mod/1 -> Discrete-Time Integrator1/3, GreaterThan/2
  Discrete-Time Integrator1/State -> GreaterThan/1, Mod/1
  w/1 -> Discrete-Time Integrator1/1  "w"
  Discrete-Time Integrator1/1 -> wt/1  "wt"
  GreaterThan/1 -> Discrete-Time Integrator1/2

== system HIL/EquivelentSimscape/Continous/abc_dqz/Subsystem ==
  abc : Inport  PortDimensions=3
  Gain1 : Gain  Gain=single(2/3)  SaturateOnIntegerOverflow=on  OutDataTypeStr=Inherit: Same as input  ParamDataTypeStr=Inherit: Same as input
  Gain3 : Gain  Gain="single([ 1   -1/2   -1/2; 0   sqrt(3)/2   -sqrt(3)/2; 1/2  1/2  1/2 ] )"  Multiplication=Matrix(K*u) (u vector)  SaturateOnIntegerOverflow=on  OutDataTypeStr=Inherit: Same as input  ParamDataTypeStr=Inherit: Same as input
  al_be_0 : Outport  VectorParamsAs1DForOutWhenUnconnected=off
  wires:
  Gain1/1 -> al_be_0/1  "AlphaBetaZero"
  Gain3/1 -> Gain1/1
  abc/1 -> Gain3/1

== system HIL/EquivelentSimscape/Continous/abc_dqz/Subsystem2 ==
  note: =
  note: *
  note: [ d
      |    q ]
  note: d = al*cos(wt) + be*sin(wt)
  note: [  cos(wt)   sin(wt)
      |    -sin(wt)    cos(wt)   ]
  note: q = -al*sin(wt) + be*cos(wt)
  note: [  al
      |     be  ]
  alpha_beta : Inport
  wtNow : Inport  Port=2  PortDimensions=1
  Fcn : Fcn  Expr=u[1]*cos(u[3]) + u[2]*sin(u[3])
  Fcn1 : Fcn  Expr=-u[1]*sin(u[3]) + u[2]*cos(u[3])
  Mux : Mux  Inputs=3
  Mux1 : Mux  Inputs=[2 1]
  Mux2 : Mux  Inputs=[2 1]
  Selector : Selector  InputPortWidth=3  IndexOptions=Index vector (dialog)  Indices=[1 2]  OutputSizes=1
  Selector1 : Selector  InputPortWidth=3  IndexOptions=Index vector (dialog)  Indices=[3]  OutputSizes=1
  dq : Outport  InitialOutput=[0,0]  VectorParamsAs1DForOutWhenUnconnected=off
  wires:
  wtNow/1 -> Mux1/2, Mux2/2
  alpha_beta/1 -> Selector/1, Selector1/1
  Mux1/1 -> Fcn/1
  Fcn1/1 -> Mux/2
  Fcn/1 -> Mux/1
  Mux/1 -> dq/1
  Mux2/1 -> Fcn1/1
  Selector/1 -> Mux2/1, Mux1/1
  Selector1/1 -> Mux/3

== system HIL/EquivelentSimscape/LGridImpedance/Subsystem1/Harmonics ==
  wt_abc : Inport
  Enable : EnablePort  StatesWhenEnabling=reset
  Cos1 : Trigonometry  Operator=cos
  Gain5 : Gain  Gain=Hil.Harm_Freq'  Multiplication=Matrix(K*u)
  Gain8 : Gain  Gain=(eye(3,3).*(Hil.Harm_Amp))  Multiplication=Matrix(K*u)
  Reshape : Reshape
  Reshape1 : Reshape  OutputDimensionality=Row vector (2-D)
  Sum of Elements : Sum  Inputs=+  CollapseMode=Specified dimension
  Harm : Outport
  wires:
  Reshape/1 -> Harm/1
  Gain8/1 -> Sum of Elements/1
  Cos1/1 -> Gain8/1
  Gain5/1 -> Cos1/1
  Reshape1/1 -> Gain5/1
  wt_abc/1 -> Reshape1/1
  Sum of Elements/1 -> Reshape/1

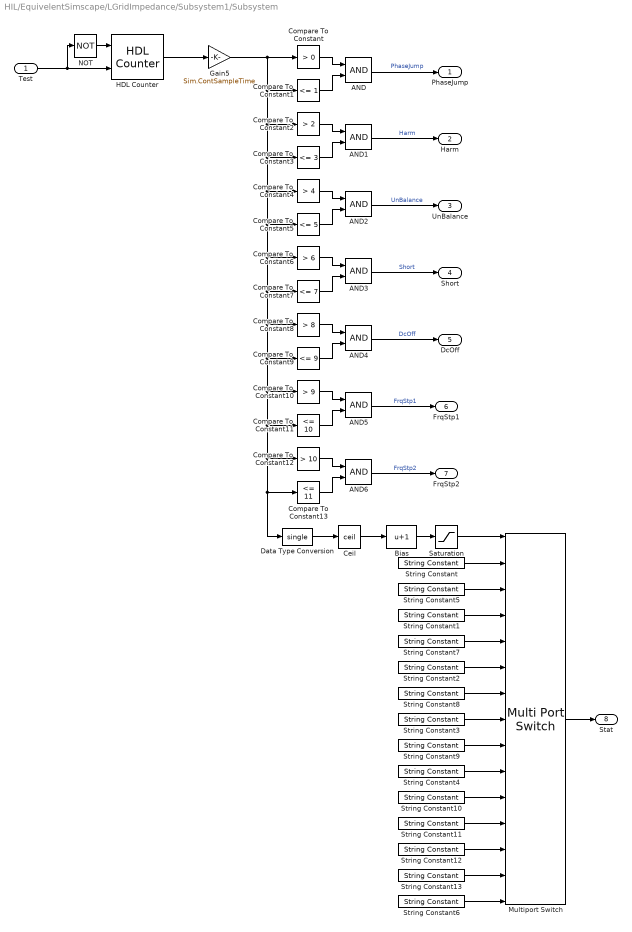
== system HIL/EquivelentSimscape/LGridImpedance/Subsystem1/Subsystem ==
  Test : Inport
  AND{,1..6} (7 alike) : Logic  AllPortsSameDT=off  OutDataTypeStr=boolean
  Bias : Bias  Bias=1  SaturateOnIntegerOverflow=off
  Ceil : Rounding  Operator=ceil
  Compare To Constant : simulink/Logic and Bit Operations/Compare To Constant  relop=>  const=0  OutDataTypeStr=boolean
  Compare To Constant1 : simulink/Logic and Bit Operations/Compare To Constant  relop=<=  const=1  OutDataTypeStr=boolean
  Compare To Constant10 : simulink/Logic and Bit Operations/Compare To Constant  relop=>  const=9  OutDataTypeStr=boolean
  Compare To Constant11 : simulink/Logic and Bit Operations/Compare To Constant  relop=<=  const=10  OutDataTypeStr=boolean
  Compare To Constant12 : simulink/Logic and Bit Operations/Compare To Constant  relop=>  const=10  OutDataTypeStr=boolean
  Compare To Constant13 : simulink/Logic and Bit Operations/Compare To Constant  relop=<=  const=11  OutDataTypeStr=boolean
  Compare To Constant2 : simulink/Logic and Bit Operations/Compare To Constant  relop=>  const=2  OutDataTypeStr=boolean
  Compare To Constant3 : simulink/Logic and Bit Operations/Compare To Constant  relop=<=  const=3  OutDataTypeStr=boolean
  Compare To Constant4 : simulink/Logic and Bit Operations/Compare To Constant  relop=>  const=4  OutDataTypeStr=boolean
  Compare To Constant5 : simulink/Logic and Bit Operations/Compare To Constant  relop=<=  const=5  OutDataTypeStr=boolean
  Compare To Constant6 : simulink/Logic and Bit Operations/Compare To Constant  relop=>  const=6  OutDataTypeStr=boolean
  Compare To Constant7 : simulink/Logic and Bit Operations/Compare To Constant  relop=<=  const=7  OutDataTypeStr=boolean
  Compare To Constant8 : simulink/Logic and Bit Operations/Compare To Constant  relop=>  const=8  OutDataTypeStr=boolean
  Compare To Constant9 : simulink/Logic and Bit Operations/Compare To Constant  relop=<=  const=9  OutDataTypeStr=boolean
  Data Type Conversion : DataTypeConversion  OutDataTypeStr=single  SaturateOnIntegerOverflow=off  RndMeth=Floor
  Gain5 : Gain  Gain=Sim.ContSampleTime  ParamDataTypeStr=double  OutDataTypeStr=double
  HDL Counter : hdlsllib/Sources/HDL Counter  CountType=Free running  CountInit=0  CountStep=1  CountMax=25  CountFromType=Initial value  CountFrom=0  CountResetPort=on  CountLoadPort=off  CountEnbPort=on  CountDirPort=off  CountHitOutputPort=off  CountDataType=Unsigned  CountWordLen=32  CountFracLen=0  CountSampTime=1
  Multiport Switch : MultiPortSwitch  Inputs=14  SaturateOnIntegerOverflow=off  InputSameDT=off
  NOT : Logic  Operator=NOT  AllPortsSameDT=off  OutDataTypeStr=boolean
  Saturation : Saturate  UpperLimit=14  LowerLimit=0
  String Constant{,1..4,6,11} (7 alike) : StringConstant  String="\"Normal\""
  String Constant10 : StringConstant  String="\"DC Offset\""
  String Constant12 : StringConstant  String="\"Freq Stp 1\""
  String Constant13 : StringConstant  String="\"Freq Stp 2\""
  String Constant5 : StringConstant  String="\"Phase Jump\""
  String Constant7 : StringConstant  String="\"Harm\""
  String Constant8 : StringConstant  String="\"Unbalance\""
  String Constant9 : StringConstant  String="\"Short\""
  PhaseJump : Outport
  Harm : Outport  Port=2
  UnBalance : Outport  Port=3
  Short : Outport  Port=4
  DcOff : Outport  Port=5
  FrqStp1 : Outport  Port=6
  FrqStp2 : Outport  Port=7
  Stat : Outport  Port=8
  wires:
  Bias/1 -> Saturation/1
  Data Type Conversion/1 -> Ceil/1
  Multiport Switch/1 -> Stat/1
  Saturation/1 -> Multiport Switch/1
  Ceil/1 -> Bias/1
  String Constant13/1 -> Multiport Switch/14
  String Constant12/1 -> Multiport Switch/13
  String Constant11/1 -> Multiport Switch/12
  String Constant10/1 -> Multiport Switch/11
  String Constant9/1 -> Multiport Switch/9
  String Constant8/1 -> Multiport Switch/7
  String Constant7/1 -> Multiport Switch/5
  String Constant5/1 -> Multiport Switch/3
  String Constant6/1 -> Multiport Switch/15
  String Constant4/1 -> Multiport Switch/10
  String Constant3/1 -> Multiport Switch/8
  String Constant2/1 -> Multiport Switch/6
  String Constant1/1 -> Multiport Switch/4
  String Constant/1 -> Multiport Switch/2
  NOT/1 -> HDL Counter/1
  Compare To Constant13/1 -> AND6/2
  Compare To Constant12/1 -> AND6/1
  AND6/1 -> FrqStp2/1  "FrqStp2"
  AND5/1 -> FrqStp1/1  "FrqStp1"
  Compare To Constant10/1 -> AND5/1
  Compare To Constant11/1 -> AND5/2
  AND/1 -> PhaseJump/1  "PhaseJump"
  Test/1 -> HDL Counter/2, NOT/1
  AND2/1 -> UnBalance/1  "UnBalance"
  AND3/1 -> Short/1  "Short"
  HDL Counter/1 -> Gain5/1
  Compare To Constant5/1 -> AND2/2
  Compare To Constant/1 -> AND/1
  Compare To Constant9/1 -> AND4/2
  Compare To Constant2/1 -> AND1/1
  Compare To Constant8/1 -> AND4/1
  Compare To Constant3/1 -> AND1/2
  AND4/1 -> DcOff/1  "DcOff"
  Compare To Constant1/1 -> AND/2
  Compare To Constant7/1 -> AND3/2
  Compare To Constant6/1 -> AND3/1
  Gain5/1 -> Compare To Constant/1, Compare To Constant1/1, Compare To Constant3/1, Compare To Constant5/1, Compare To Constant7/1, Compare To Constant8/1, Compare To Constant9/1, Compare To Constant13/1, Data Type Conversion/1, Compare To Constant12/1, Compare To Constant11/1, Compare To Constant10/1, Compare To Constant6/1, Compare To Constant4/1, Compare To Constant2/1
  AND1/1 -> Harm/1  "Harm"
  Compare To Constant4/1 -> AND2/1

== system HIL/EquivelentSimscape/LGridImpedance/Subsystem1/WrappedIntegrator ==
  w : Inport
  Constant1 : Constant  Value=2*pi
  Discrete-Time Integrator1 : DiscreteIntegrator  gainval=single(1)  ExternalReset=rising  InitialConditionSource=external  SampleTime=-1  ShowStatePort=on  ICPrevOutput=DiscIntNeverNeededParam  ICPrevScaledInput=DiscIntNeverNeededParam
  GreaterThan : RelationalOperator  Operator=~=  OutDataTypeStr=boolean  RndMeth=Simplest  InputSameDT=off
  Mod : Math  Operator=mod
  wt : Outport
  wires:
  GreaterThan/1 -> Discrete-Time Integrator1/2
  Discrete-Time Integrator1/1 -> wt/1  "wt"
  w/1 -> Discrete-Time Integrator1/1
  Discrete-Time Integrator1/State -> Mod/1, GreaterThan/1
  Mod/1 -> GreaterThan/2, Discrete-Time Integrator1/3
  Constant1/1 -> Mod/2

== system HIL/EquivelentSimscape/Taraz/Subsystem2/Harmonics ==
  wt_abc : Inport
  Enable : EnablePort  StatesWhenEnabling=reset
  Cos1 : Trigonometry  Operator=cos
  Gain5 : Gain  Gain=Hil.Harm_Freq'  Multiplication=Matrix(K*u)
  Gain8 : Gain  Gain=(eye(3,3).*(Hil.Harm_Amp))  Multiplication=Matrix(K*u)
  Reshape : Reshape
  Reshape1 : Reshape  OutputDimensionality=Row vector (2-D)
  Sum of Elements : Sum  Inputs=+  CollapseMode=Specified dimension
  Harm : Outport
  wires:
  Reshape/1 -> Harm/1
  Gain8/1 -> Sum of Elements/1
  Cos1/1 -> Gain8/1
  Gain5/1 -> Cos1/1
  Reshape1/1 -> Gain5/1
  wt_abc/1 -> Reshape1/1
  Sum of Elements/1 -> Reshape/1

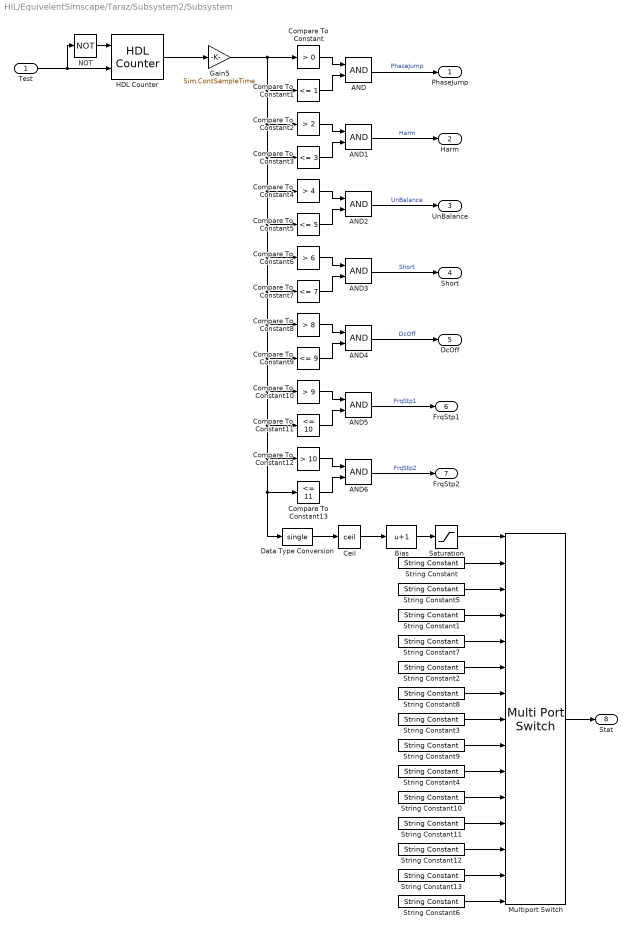
== system HIL/EquivelentSimscape/Taraz/Subsystem2/Subsystem ==
  Test : Inport
  AND{,1..6} (7 alike) : Logic  AllPortsSameDT=off  OutDataTypeStr=boolean
  Bias : Bias  Bias=1  SaturateOnIntegerOverflow=off
  Ceil : Rounding  Operator=ceil
  Compare To Constant : simulink/Logic and Bit Operations/Compare To Constant  relop=>  const=0  OutDataTypeStr=boolean
  Compare To Constant1 : simulink/Logic and Bit Operations/Compare To Constant  relop=<=  const=1  OutDataTypeStr=boolean
  Compare To Constant10 : simulink/Logic and Bit Operations/Compare To Constant  relop=>  const=9  OutDataTypeStr=boolean
  Compare To Constant11 : simulink/Logic and Bit Operations/Compare To Constant  relop=<=  const=10  OutDataTypeStr=boolean
  Compare To Constant12 : simulink/Logic and Bit Operations/Compare To Constant  relop=>  const=10  OutDataTypeStr=boolean
  Compare To Constant13 : simulink/Logic and Bit Operations/Compare To Constant  relop=<=  const=11  OutDataTypeStr=boolean
  Compare To Constant2 : simulink/Logic and Bit Operations/Compare To Constant  relop=>  const=2  OutDataTypeStr=boolean
  Compare To Constant3 : simulink/Logic and Bit Operations/Compare To Constant  relop=<=  const=3  OutDataTypeStr=boolean
  Compare To Constant4 : simulink/Logic and Bit Operations/Compare To Constant  relop=>  const=4  OutDataTypeStr=boolean
  Compare To Constant5 : simulink/Logic and Bit Operations/Compare To Constant  relop=<=  const=5  OutDataTypeStr=boolean
  Compare To Constant6 : simulink/Logic and Bit Operations/Compare To Constant  relop=>  const=6  OutDataTypeStr=boolean
  Compare To Constant7 : simulink/Logic and Bit Operations/Compare To Constant  relop=<=  const=7  OutDataTypeStr=boolean
  Compare To Constant8 : simulink/Logic and Bit Operations/Compare To Constant  relop=>  const=8  OutDataTypeStr=boolean
  Compare To Constant9 : simulink/Logic and Bit Operations/Compare To Constant  relop=<=  const=9  OutDataTypeStr=boolean
  Data Type Conversion : DataTypeConversion  OutDataTypeStr=single  SaturateOnIntegerOverflow=off  RndMeth=Floor
  Gain5 : Gain  Gain=Sim.ContSampleTime  ParamDataTypeStr=double  OutDataTypeStr=double
  HDL Counter : hdlsllib/Sources/HDL Counter  CountType=Free running  CountInit=0  CountStep=1  CountMax=25  CountFromType=Initial value  CountFrom=0  CountResetPort=on  CountLoadPort=off  CountEnbPort=on  CountDirPort=off  CountHitOutputPort=off  CountDataType=Unsigned  CountWordLen=32  CountFracLen=0  CountSampTime=1
  Multiport Switch : MultiPortSwitch  Inputs=14  SaturateOnIntegerOverflow=off  InputSameDT=off
  NOT : Logic  Operator=NOT  AllPortsSameDT=off  OutDataTypeStr=boolean
  Saturation : Saturate  UpperLimit=14  LowerLimit=0
  String Constant{,1..4,6,11} (7 alike) : StringConstant  String="\"Normal\""
  String Constant10 : StringConstant  String="\"DC Offset\""
  String Constant12 : StringConstant  String="\"Freq Stp 1\""
  String Constant13 : StringConstant  String="\"Freq Stp 2\""
  String Constant5 : StringConstant  String="\"Phase Jump\""
  String Constant7 : StringConstant  String="\"Harm\""
  String Constant8 : StringConstant  String="\"Unbalance\""
  String Constant9 : StringConstant  String="\"Short\""
  PhaseJump : Outport
  Harm : Outport  Port=2
  UnBalance : Outport  Port=3
  Short : Outport  Port=4
  DcOff : Outport  Port=5
  FrqStp1 : Outport  Port=6
  FrqStp2 : Outport  Port=7
  Stat : Outport  Port=8
  wires:
  Bias/1 -> Saturation/1
  Data Type Conversion/1 -> Ceil/1
  Multiport Switch/1 -> Stat/1
  Saturation/1 -> Multiport Switch/1
  Ceil/1 -> Bias/1
  String Constant13/1 -> Multiport Switch/14
  String Constant12/1 -> Multiport Switch/13
  String Constant11/1 -> Multiport Switch/12
  String Constant10/1 -> Multiport Switch/11
  String Constant9/1 -> Multiport Switch/9
  String Constant8/1 -> Multiport Switch/7
  String Constant7/1 -> Multiport Switch/5
  String Constant5/1 -> Multiport Switch/3
  String Constant6/1 -> Multiport Switch/15
  String Constant4/1 -> Multiport Switch/10
  String Constant3/1 -> Multiport Switch/8
  String Constant2/1 -> Multiport Switch/6
  String Constant1/1 -> Multiport Switch/4
  String Constant/1 -> Multiport Switch/2
  NOT/1 -> HDL Counter/1
  Compare To Constant13/1 -> AND6/2
  Compare To Constant12/1 -> AND6/1
  AND6/1 -> FrqStp2/1  "FrqStp2"
  AND5/1 -> FrqStp1/1  "FrqStp1"
  Compare To Constant10/1 -> AND5/1
  Compare To Constant11/1 -> AND5/2
  AND/1 -> PhaseJump/1  "PhaseJump"
  Test/1 -> HDL Counter/2, NOT/1
  AND2/1 -> UnBalance/1  "UnBalance"
  AND3/1 -> Short/1  "Short"
  HDL Counter/1 -> Gain5/1
  Compare To Constant5/1 -> AND2/2
  Compare To Constant/1 -> AND/1
  Compare To Constant9/1 -> AND4/2
  Compare To Constant2/1 -> AND1/1
  Compare To Constant8/1 -> AND4/1
  Compare To Constant3/1 -> AND1/2
  AND4/1 -> DcOff/1  "DcOff"
  Compare To Constant1/1 -> AND/2
  Compare To Constant7/1 -> AND3/2
  Compare To Constant6/1 -> AND3/1
  Gain5/1 -> Compare To Constant/1, Compare To Constant1/1, Compare To Constant3/1, Compare To Constant5/1, Compare To Constant7/1, Compare To Constant8/1, Compare To Constant9/1, Compare To Constant13/1, Data Type Conversion/1, Compare To Constant12/1, Compare To Constant11/1, Compare To Constant10/1, Compare To Constant6/1, Compare To Constant4/1, Compare To Constant2/1
  AND1/1 -> Harm/1  "Harm"
  Compare To Constant4/1 -> AND2/1

== system HIL/EquivelentSimscape/Taraz/Subsystem2/WrappedIntegrator ==
  w : Inport
  Constant1 : Constant  Value=2*pi
  Discrete-Time Integrator1 : DiscreteIntegrator  gainval=single(1)  ExternalReset=rising  InitialConditionSource=external  SampleTime=-1  ShowStatePort=on  ICPrevOutput=DiscIntNeverNeededParam  ICPrevScaledInput=DiscIntNeverNeededParam
  GreaterThan : RelationalOperator  Operator=~=  OutDataTypeStr=boolean  RndMeth=Simplest  InputSameDT=off
  Mod : Math  Operator=mod
  wt : Outport
  wires:
  GreaterThan/1 -> Discrete-Time Integrator1/2
  Discrete-Time Integrator1/1 -> wt/1  "wt"
  w/1 -> Discrete-Time Integrator1/1
  Discrete-Time Integrator1/State -> Mod/1, GreaterThan/1
  Mod/1 -> GreaterThan/2, Discrete-Time Integrator1/3
  Constant1/1 -> Mod/2

== system HIL/EquivelentSimscape/TarazAvg/Subsystem1/Harmonics ==
  wt_abc : Inport
  Enable : EnablePort  StatesWhenEnabling=reset
  Cos1 : Trigonometry  Operator=cos
  Gain5 : Gain  Gain=Hil.Harm_Freq'  Multiplication=Matrix(K*u)
  Gain8 : Gain  Gain=(eye(3,3).*(Hil.Harm_Amp))  Multiplication=Matrix(K*u)
  Reshape : Reshape
  Reshape1 : Reshape  OutputDimensionality=Row vector (2-D)
  Sum of Elements : Sum  Inputs=+  CollapseMode=Specified dimension
  Harm : Outport
  wires:
  Reshape/1 -> Harm/1
  Gain8/1 -> Sum of Elements/1
  Cos1/1 -> Gain8/1
  Gain5/1 -> Cos1/1
  Reshape1/1 -> Gain5/1
  wt_abc/1 -> Reshape1/1
  Sum of Elements/1 -> Reshape/1
